simulink model "MODEL_with_panthera"  (R2019b)
settings: Solver=ode1  StartTime=0.0  StopTime=inf  FixedStep=0.001  RelTol=1e-3  EnableMultiTasking=on
PreLoadFcn:
  | run('m-files/add_to_path.m')
InitFcn:
  | create_ephysenet_inifile
undefined symbols (not defined in the file or in its folder): car
libraries: realtime_pacer_lib x2, ephysenetlib x2, car_library x1
CloseFcn:
  | delete_ephysenet_inifile
settings Model: Creator=ciba  LastModifiedBy=LongLongMagnumDong
settings SolverCC: AutoInsertRateTranBlk=on
settings DataIOCC: LimitDataPoints=on  SaveFormat=Structure  SaveState=on  SignalLogging=off  ReturnWorkspaceOutputs=off
settings OptimizationCC: LifeSpan=inf
settings DebuggingCC: SolverPrmCheckMsg=warning  SFUnexpectedBacktrackingDiag=warning  SFNoUnconditionalDefaultTransitionDiag=warning  SFExecutionAtInitializationDiag=none  ArithmeticOperatorsInVariantConditions=warning
settings HardwareCC: ProdBitPerPointer=32  ProdBitPerSizeT=32  ProdBitPerPtrDiffT=32  ProdLargestAtomicFloat=None  ProdIntDivRoundTo=Undefined  ProdEndianess=Unspecified  ProdWordSize=32  ProdHWDeviceType=32-bit Generic
settings ModelReferenceCC: PropagateSignalLabelsOutOfModel=off
settings SFSimCC: SimUseLocalCustomCode=off  CustomCodeUndefinedFunction=UseInterfaceOnly
settings RTWCC: RTWUseLocalCustomCode=off
settings CodeAppCC: StateflowObjectComments=on
settings GRTTargetCC: TargetLangStandard=C89/C90 (ANSI)  GeneratePreprocessorConditionals=Disable all
settings ConfigComp: CovMetricSettings=dw  CovHtmlReporting=on  CovSaveCumulativeToWorkspaceVar=on  CovSaveSingleToWorkspaceVar=on  CovExternalEMLEnable=off

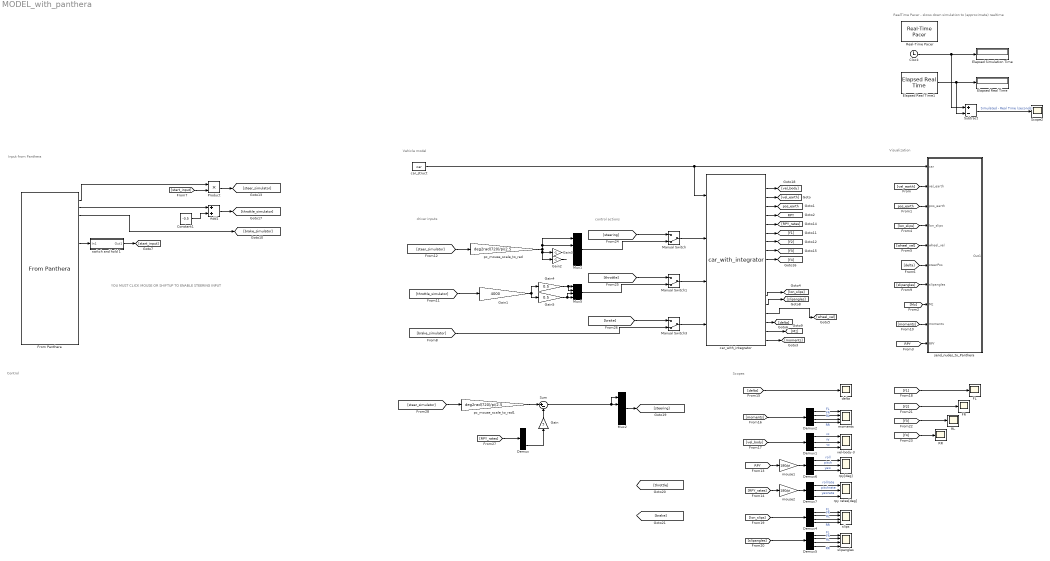
== system MODEL_with_panthera ==
  note: driver inputs
  note: control actions
  note: Control
  note: Scopes
  note: RealTime Pacer - slows down simulation to (approximate) realtime
  note: Visualization
  note: Vehicle model
  note: Input from Panthera
  note: YOU MUST CLICK MOUSE OR SHIFTUP
      | TO ENABLE STEERING INPUT
  Add1 : Sum
  Clock : Clock
  Constant1 : Constant  Value=-0.5
  Demux{,1,6..7} (4 alike) : Demux  Outputs=3
  Demux2 : Demux
  Demux4 : Demux
  Demux5 : Demux
  Elapsed Real Time : Display
      settings: Decimation=2
  Elapsed Real Time1 : realtime_pacer_lib/Elapsed Real Time
  Elapsed Simulation Time : Display
      settings: Decimation=2
  FL : Scope
  FR : Scope
  From Panthera : ephysenetlib/Input blocks/From Panthera
  Gain : Gain  Gain=5
  Gain1 : Gain  Gain=4000
  Gain2 : Gain  Gain=-1
  Gain3 : Gain  Gain=-1
  Gain4 : Gain  Gain=0.5
  Gain5 : Gain  Gain=0.5
  Manual Switch : ManualSwitch  CurrentSetting=0
  Manual Switch1 : ManualSwitch  CurrentSetting=0
  Manual Switch3 : ManualSwitch  CurrentSetting=0
  Mux1 : Mux
  Mux2 : Mux
  Mux5 : Mux
  Product : Product
  RL : Scope
  RR : Scope
  Real-Time Pacer : realtime_pacer_lib/Real-Time Pacer  simTimePerRealTime=1
  Scope2 : Scope
  Subtract : Sum  Inputs=+-
  Sum : Sum  Inputs=|+-
  car_struct : Constant  Value=car  OutDataTypeStr=Bus: car_bus
  car_with_integrator : car_library/car_with_integrator  SystemSampleTime=-1  Latency=0  AutoFrameSizeCalculation=off
      link override Constant2: Value=[1;1;1;1]
  delta : Scope
  moments : Scope  NumInputPorts=4
  mouse1 : Gain  Gain=180/pi
  mouse2 : Gain  Gain=180/pi
  pc_mouse_scale_to_rad : Gain  Gain=deg2rad(720)/pi/2.5
  pc_mouse_scale_to_rad1 : Gain  Gain=deg2rad(720)/pi/2.5
  rpy rates[deg] : Scope  NumInputPorts=3
  "rpy[deg] " : Scope  NumInputPorts=3
  send_nudes_to_Panthera : Subsystem
  slipangles : Scope  NumInputPorts=4
  slips : Scope  NumInputPorts=4
  switch and hold 1 : Subsystem
  "vel-body-3 " : Scope  NumInputPorts=3
  tag scope: RPY=global, pos_earth=global
  wires:
  car_with_integrator/3 -> [vel_earth]
  [vel_earth] -> send_nudes_to_Panthera/2(vel_earth)
  car_with_integrator/4 -> [pos_earth]
  car_with_integrator/16 -> [wheel_vel]
  [pos_earth] -> send_nudes_to_Panthera/3(pos_earth)
  [lon_slips] -> send_nudes_to_Panthera/4(lon_slips)
  [wheel_vel] -> send_nudes_to_Panthera/5(wheel_vel)
  [delta] -> send_nudes_to_Panthera/6(steerPos)
  Clock/1 -> Elapsed Simulation Time/1, Subtract/1
  Subtract/1 -> Scope2/1  "Simulated - Real Time (seconds)"
  Elapsed Real Time1/1 -> Elapsed Real Time/1, Subtract/2
  car_with_integrator/15 -> [slipangles]
  car_with_integrator/5 -> [RPY]
  From Panthera/3 -> [brake_simulator]
  [slipangles] -> send_nudes_to_Panthera/7(slipangles)
  From Panthera/7 -> switch and hold 1/1(In1)
  [RPY] -> send_nudes_to_Panthera/10("RPY ")
  [moments] -> send_nudes_to_Panthera/9(moments)
  car_with_integrator/19 -> [moments]
  From Panthera/1 -> Product/1
  [start_input] -> Product/2
  Product/1 -> [steer_simulator]
  From Panthera/2 -> Add1/1
  Constant1/1 -> Add1/2
  car_with_integrator/17 -> [delta]
  [RPY] -> mouse1/1
  [delta] -> delta/1
  car_with_integrator/6 -> [RPY_rates]
  [moments] -> Demux2/1
  Demux2/1 -> moments/1  "FL"
  Demux2/2 -> moments/2  "FR"
  Demux2/3 -> moments/3  "RL"
  Demux2/4 -> moments/4  "RR"
  Demux4/1 -> slips/1  "FL"
  Demux4/2 -> slips/2  "FR"
  Demux4/3 -> slips/3  "RL"
  Demux4/4 -> slips/4  "RR"
  [lon_slips] -> Demux4/1
  Demux5/1 -> slipangles/1  "FL"
  Demux5/2 -> slipangles/2  "FR"
  Demux5/3 -> slipangles/3  "RL"
  Demux5/4 -> slipangles/4  "RR"
  [slipangles] -> Demux5/1
  car_with_integrator/14 -> [lon_slips]
  car_with_integrator/18 -> [Mz]
  [Mz] -> send_nudes_to_Panthera/8(Mz)
  switch and hold 1/1(Out1) -> [start_input]
  car_with_integrator/7 -> [f1]
  car_with_integrator/8 -> [f2]
  car_with_integrator/9 -> [f3]
  car_with_integrator/10 -> [f4]
  Add1/1 -> [throttle_simulator]
  pc_mouse_scale_to_rad/1 -> Mux1/2, Mux1/1, Gain2/1, Gain3/1
  Manual Switch1/1 -> car_with_integrator/3
  Mux5/1 -> Manual Switch1/2
  [steer_simulator] -> pc_mouse_scale_to_rad/1
  Gain1/1 -> Gain4/1, Gain5/1
  Gain5/1 -> Mux5/4, Mux5/3
  Gain4/1 -> Mux5/2, Mux5/1
  car_struct/1 -> car_with_integrator/1, send_nudes_to_Panthera/1(car)
  Gain2/1 -> ?
  Gain3/1 -> ?
  [brake_simulator] -> Manual Switch3/2
  car_with_integrator/2 -> [vel_body]
  [vel_body] -> Demux1/1
  Demux1/2 -> "vel-body-3 "/2  "vy"
  Demux1/1 -> "vel-body-3 "/1  "vx"
  Demux1/3 -> "vel-body-3 "/3  "vz"
  [throttle_simulator] -> Gain1/1
  Manual Switch3/1 -> car_with_integrator/4
  [brake] -> Manual Switch3/1
  [throttle] -> Manual Switch1/1
  [steering] -> Manual Switch/1
  Manual Switch/1 -> car_with_integrator/2
  Mux1/1 -> Manual Switch/2
  mouse1/1 -> Demux6/1
  Demux6/1 -> "rpy[deg] "/1  "roll"
  Demux6/2 -> "rpy[deg] "/2  "pitch"
  Demux6/3 -> "rpy[deg] "/3  "yaw"
  Demux7/3 -> rpy rates[deg]/3  "yawrate"
  Demux7/2 -> rpy rates[deg]/2  "pitchrate"
  [RPY_rates] -> mouse2/1
  mouse2/1 -> Demux7/1
  Demux7/1 -> rpy rates[deg]/1  "rollrate"
  [f1] -> FL/1
  [f2] -> FR/1
  [f3] -> RL/1
  [f4] -> RR/1
  [RPY_rates] -> Demux/1
  [steer_simulator] -> pc_mouse_scale_to_rad1/1
  pc_mouse_scale_to_rad1/1 -> Sum/1
  Demux/3 -> Gain/1
  Gain/1 -> Sum/2
  Sum/1 -> Mux2/1, Mux2/2
  Mux2/1 -> [steering]

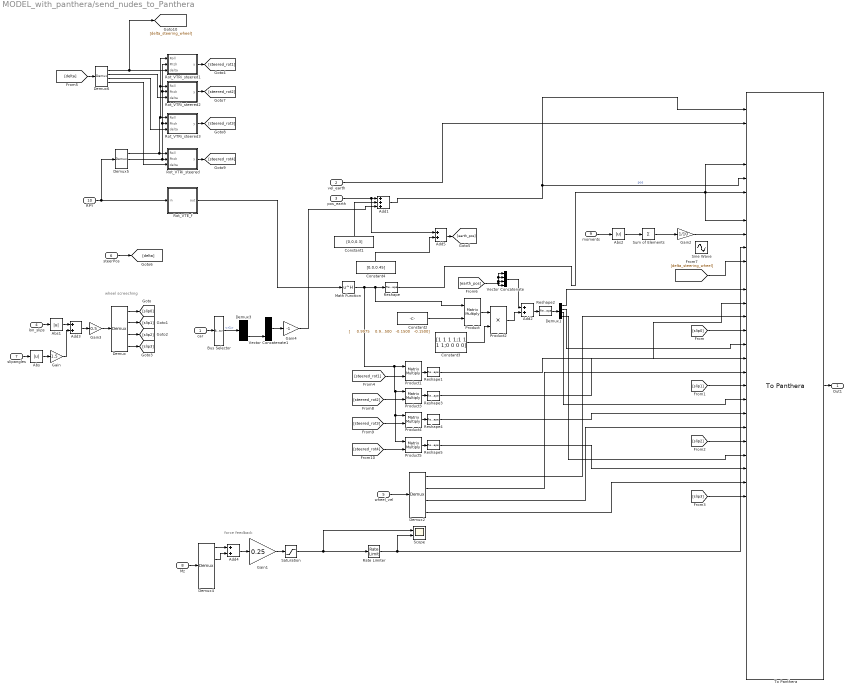
== system MODEL_with_panthera/send_nudes_to_Panthera ==
  note: force feedback
  note: wheel screeching
  car : Inport
  vel_earth : Inport  Port=2
  pos_earth : Inport  Port=3
  lon_slips : Inport  Port=4
  wheel_vel : Inport  Port=5
  steerPos : Inport  Port=6
  slipangles : Inport  Port=7
  Mz : Inport  Port=8
  moments : Inport  Port=9
  "RPY " : Inport  Port=10
  Abs : Abs
  Abs1 : Abs
  Abs2 : Abs
  Add1 : Sum  Inputs=+++
  Add{2..5} (4 alike) : Sum
  Bus Selector : BusSelector  OutputSignals=r1
  Constant1 : Constant  Value=[0,0,0.3]
  Constant2 : Constant  Value=|
      | [
      |     0.9975    0.9975   -1.7475   -1.7475;
      |     0.8500   -0.8500    0.8500   -0.8500;
      |    -0.1500   -0.1500   -0.1500   -0.1500]
  Constant3 : Constant  Value=[1 1 1 1;1 1 1 1;0 0 0 0]
  Constant4 : Constant  Value=[0,0,0.45]
  Demux{,1..2,4,6} (5 alike) : Demux
  Demux3 : Demux  Outputs=3
  Demux5 : Demux  Outputs=3
  Gain : Gain  Gain=1.5
  Gain1 : Gain  Gain=0.25
  Gain2 : Gain  Gain=1/10
  Gain3 : Gain  Gain=0.5
  Gain4 : Gain  Gain=-1
  Math Function : Math  Operator=hermitian  SaturateOnIntegerOverflow=on
  Product{,1,3..5} (5 alike) : Product  Multiplication=Matrix(*)
  Product2 : Product
  Rate Limiter : RateLimiter  RisingSlewLimit=500  FallingSlewLimit=-500  SampleTimeMode=inherited
  Reshape{,1,3..5} (5 alike) : Reshape
  Reshape2 : Reshape  OutputDimensionality=Customize  OutputDimensions=[1,12]
  Rot_VTE_f : MATLAB Function  TreatAsAtomicUnit=on
  Rot_VTRi_steered : MATLAB Function  TreatAsAtomicUnit=on
  Rot_VTRi_steered1 : MATLAB Function  TreatAsAtomicUnit=on
  Rot_VTRi_steered2 : MATLAB Function  TreatAsAtomicUnit=on
  Rot_VTRi_steered3 : MATLAB Function  TreatAsAtomicUnit=on
  Saturation : Saturate  UpperLimit=200  LowerLimit=-200
  Scope : Scope  NumInputPorts=2
  Sine Wave : Sin  Amplitude=1000  Frequency=0.1  SampleTime=0
  Sum of Elements : Sum  Inputs=+
  To Panthera : ephysenetlib/Output blocks/To Panthera
  Vector Concatenate : Concatenate  NumInputs=4  Mode=Multidimensional array  ConcatenateDimension=2
  Vector Concatenate1 : Concatenate  NumInputs=3
  Out1 : Outport  VectorParamsAs1DForOutWhenUnconnected=off
  wires:
  To Panthera/1 -> Out1/1
  ? -> To Panthera/3
  ? -> To Panthera/4
  ? -> To Panthera/8
  Rot_VTE_f/1(out) -> Math Function/1
  Math Function/1 -> Product/1, Reshape/1, Product5/1, Product4/1, Product3/1, Product1/1
  pos_earth/1 -> Add5/1, Add1/1
  Constant1/1 -> Add1/2
  Demux/1 -> [slip0]
  Demux/2 -> [slip1]
  Demux/3 -> [slip2]
  Demux/4 -> [slip3]
  [slip0] -> To Panthera/17
  [slip1] -> To Panthera/21
  [slip2] -> To Panthera/25
  [slip3] -> To Panthera/29
  Rot_VTRi_steered/1(y) -> [steered_rot4]
  Constant2/1 -> Product/2
  Vector Concatenate/1 -> Add2/1
  [earth_pos] -> Vector Concatenate/4, Vector Concatenate/1, Vector Concatenate/2, Vector Concatenate/3
  Add2/1 -> Reshape2/1
  Reshape2/1 -> Demux1/1
  Demux1/1 -> To Panthera/14
  Demux1/2 -> To Panthera/18
  Demux1/3 -> To Panthera/22
  Demux1/4 -> To Panthera/26
  [steered_rot1] -> Product1/2
  Product1/1 -> Reshape1/1
  Reshape1/1 -> To Panthera/15
  Reshape/1 -> To Panthera/9, To Panthera/5, To Panthera/7
  Add1/1 -> To Panthera/6, To Panthera/1  "pos"
  Product/1 -> Product2/1
  Product2/1 -> Add2/2
  Constant3/1 -> Product2/2
  Add3/1 -> Gain3/1
  wheel_vel/1 -> Demux2/1
  Demux2/1 -> To Panthera/16
  Demux2/2 -> To Panthera/20
  Demux2/3 -> To Panthera/24
  Demux2/4 -> To Panthera/28
  steerPos/1 -> [delta]
  slipangles/1 -> Abs/1
  lon_slips/1 -> Abs1/1
  Abs/1 -> Gain/1
  Abs1/1 -> Add3/1
  Gain/1 -> Add3/2
  Mz/1 -> Demux4/1
  Demux4/1 -> Add4/1
  Demux4/2 -> Add4/2
  Add4/1 -> Gain1/1
  Gain1/1 -> Saturation/1
  Saturation/1 -> Rate Limiter/1, Scope/1
  moments/1 -> Abs2/1
  "RPY "/1 -> Demux5/1, Rot_VTE_f/1(in)
  Demux5/1 -> Rot_VTRi_steered1/1(Roll), Rot_VTRi_steered2/1(Roll), Rot_VTRi_steered3/1(Roll), Rot_VTRi_steered/1(Roll)
  Demux5/2 -> Rot_VTRi_steered1/2(Pitch), Rot_VTRi_steered2/2(Pitch), Rot_VTRi_steered3/2(Pitch), Rot_VTRi_steered/2(Pitch)
  [delta_steering_wheel] -> To Panthera/12
  vel_earth/1 -> To Panthera/2
  Sum of Elements/1 -> Gain2/1
  Gain2/1 -> To Panthera/10
  Abs2/1 -> Sum of Elements/1
  Rate Limiter/1 -> Scope/2, To Panthera/11
  Gain3/1 -> Demux/1
  car/1 -> Bus Selector/1
  Bus Selector/1 -> Demux3/1  "<r1>"
  Vector Concatenate1/1 -> Gain4/1
  Add5/1 -> [earth_pos]
  Constant4/1 -> Add5/2
  Demux3/3 -> Vector Concatenate1/3
  Gain4/1 -> Add1/3
  [delta] -> Demux6/1
  Demux6/1 -> [delta_steering_wheel], Rot_VTRi_steered1/3(delta)
  Demux6/2 -> Rot_VTRi_steered2/3(delta)
  Demux6/3 -> Rot_VTRi_steered3/3(delta)
  Demux6/4 -> Rot_VTRi_steered/3(delta)
  Rot_VTRi_steered1/1(y) -> [steered_rot1]
  Rot_VTRi_steered2/1(y) -> [steered_rot2]
  Rot_VTRi_steered3/1(y) -> [steered_rot3]
  Product3/1 -> Reshape3/1
  Product4/1 -> Reshape4/1
  Product5/1 -> Reshape5/1
  [steered_rot4] -> Product5/2
  [steered_rot3] -> Product4/2
  [steered_rot2] -> Product3/2
  Reshape3/1 -> To Panthera/19
  Reshape4/1 -> To Panthera/23
  Reshape5/1 -> To Panthera/27

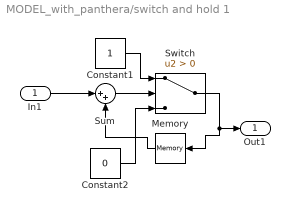
== system MODEL_with_panthera/switch and hold 1 ==
  In1 : Inport
  Constant1 : Constant
  Constant2 : Constant  Value=0
  Memory : Memory
  Sum : Sum  Inputs=|++
  Switch : Switch  Criteria=u2 > Threshold
  Out1 : Outport  VectorParamsAs1DForOutWhenUnconnected=off
  wires:
  Constant2/1 -> Switch/3
  In1/1 -> Sum/1
  Memory/1 -> Sum/2
  Constant1/1 -> Switch/1
  Sum/1 -> Switch/2
  Switch/1 -> Out1/1, Memory/1

== matlab function MODEL_with_panthera/send_nudes_to_Panthera/Rot_VTRi_steered1 ==
  data: Roll input; y output; Pitch input; delta input
function y = fcn(Roll,Pitch,delta)
y = Rot_RiTV(Roll,Pitch,delta)';

== matlab function MODEL_with_panthera/send_nudes_to_Panthera/Rot_VTRi_steered2 ==
  data: Roll input; y output; Pitch input; delta input
function y = fcn(Roll,Pitch,delta)
y = Rot_RiTV(Roll,Pitch,delta)';

== matlab function MODEL_with_panthera/send_nudes_to_Panthera/Rot_VTRi_steered3 ==
  data: Roll input; y output; Pitch input; delta input
function y = fcn(Roll,Pitch,delta)
y = Rot_RiTV(Roll,Pitch,delta)';

== matlab function MODEL_with_panthera/send_nudes_to_Panthera/Rot_VTE_f ==
  data: in input; out output
function out   = fcn(in)
out = Rot_VTE(in);

== matlab function MODEL_with_panthera/send_nudes_to_Panthera/Rot_VTRi_steered ==
  data: Roll input; y output; Pitch input; delta input
function y = fcn(Roll,Pitch,delta)
y = Rot_RiTV(Roll,Pitch,delta)';
